simulink model "prob9"  (R2020a)
settings: Solver=VariableStepAuto  StartTime=0.0  StopTime=10  RelTol=1e-3
values from neighbouring files (symbols this model uses):
  J = 1.8395E-5    [data.sldd]    (also in para.m = 1.8395e-05)
  kf = 0.0001    [data.sldd]    (also in para.m)
  Te = 100.0    [data.sldd]    (also in para.m = 100)
  TL = 50.0    [data.sldd]    (also in para.m = 50)
settings Model: DataDictionary=data.sldd  Creator=vijay  LastModifiedBy=vijay

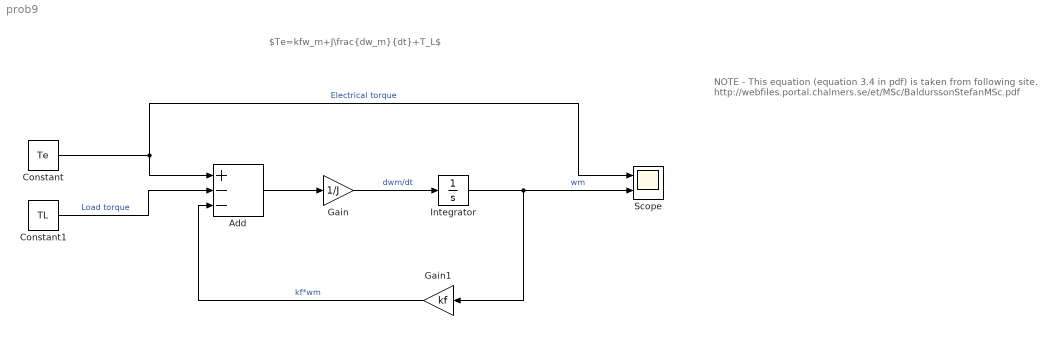
== system prob9 ==
  note: NOTE -
      |
      | This equation (equation 3.4 in pdf) is taken from following site.
      |
      | http://webfiles.portal.chalmers.se/et/MSc/BaldurssonStefanMSc.pdf
  note: $Te=kfw_m+J\frac{dw_m}{dt}+T_L$
  Add : Sum  Inputs=+--
  Constant : Constant  Value=Te
  Constant1 : Constant  Value=TL
  Gain : Gain  Gain=1/J
  Gain1 : Gain  Gain=kf
  Integrator : Integrator
  Scope : Scope  NumInputPorts=2
  wires:
  Constant1/1 -> Add/2  "Load torque"
  Gain/1 -> Integrator/1  "dwm/dt"
  Add/1 -> Gain/1
  Integrator/1 -> Gain1/1, Scope/2  "wm"
  Gain1/1 -> Add/3  "kf*wm"
  Constant/1 -> Scope/1, Add/1  "Electrical torque"
